simulink model "a3"  (R2021b)
settings: Solver=VariableStepAuto  StartTime=0.0  StopTime=500  RelTol=1e-3
libraries: simulink_extras x3
settings Model: Creator=郭义月  LastModifiedBy=郭义月

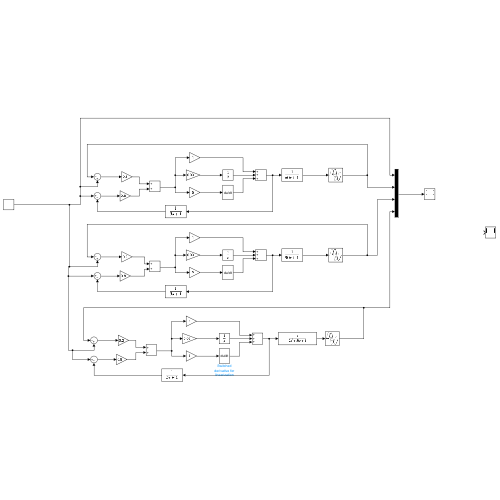
[thumbnail: Simulink's stored preview of the top-level diagram]
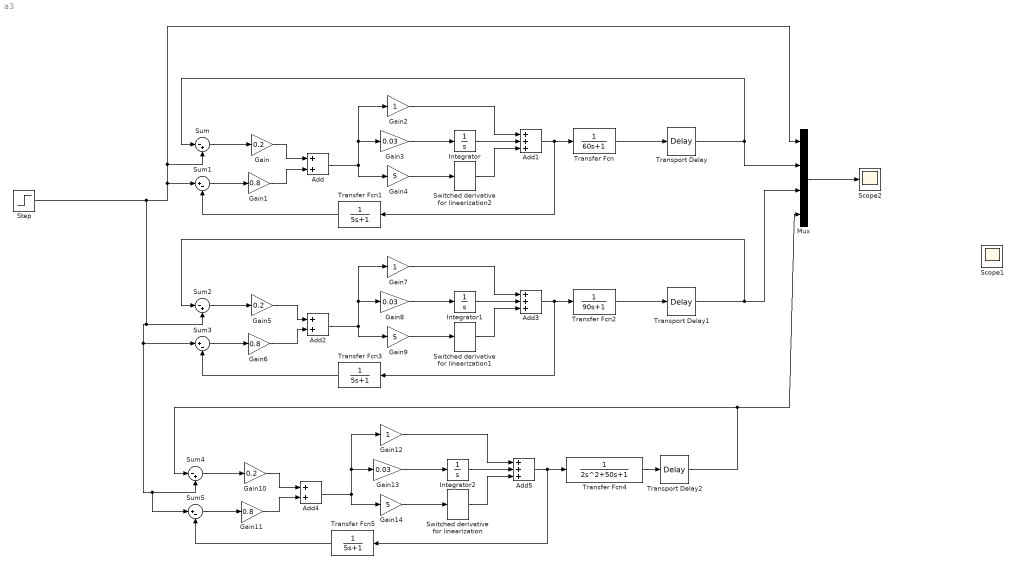
== system a3 ==
  Add : Sum
  Add1 : Sum  Inputs=+++
  Add2 : Sum
  Add3 : Sum  Inputs=+++
  Add4 : Sum
  Add5 : Sum  Inputs=+++
  Gain : Gain  Gain=0.2
  Gain1 : Gain  Gain=0.8
  Gain10 : Gain  Gain=0.2
  Gain11 : Gain  Gain=0.8
  Gain12 : Gain
  Gain13 : Gain  Gain=0.03
  Gain14 : Gain  Gain=5
  Gain2 : Gain
  Gain3 : Gain  Gain=0.03
  Gain4 : Gain  Gain=5
  Gain5 : Gain  Gain=0.2
  Gain6 : Gain  Gain=0.8
  Gain7 : Gain
  Gain8 : Gain  Gain=0.03
  Gain9 : Gain  Gain=5
  Integrator : Integrator
  Integrator1 : Integrator
  Integrator2 : Integrator
  Mux : Mux
  Scope1 : Scope
  Scope2 : Scope
  Step : Step  SampleTime=0
  Sum : Sum  Inputs=|-+
  Sum1 : Sum  Inputs=|+-
  Sum2 : Sum  Inputs=|-+
  Sum3 : Sum  Inputs=|+-
  Sum4 : Sum  Inputs=|-+
  Sum5 : Sum  Inputs=|+-
  Switched derivative for linearization : simulink_extras/Linearization/Switched derivative for linearization  switchVal=0  derivConst=100
      settings: SourceProductBaseCode=SL
  Switched derivative for linearization1 : simulink_extras/Linearization/Switched derivative for linearization  switchVal=0  derivConst=100
      settings: SourceProductBaseCode=SL
  Switched derivative for linearization2 : simulink_extras/Linearization/Switched derivative for linearization  switchVal=0  derivConst=100
      settings: SourceProductBaseCode=SL
  Transfer Fcn : TransferFcn  Denominator=[60 1]
  Transfer Fcn1 : TransferFcn  Denominator=[5 1]
  Transfer Fcn2 : TransferFcn  Denominator=[90 1]
  Transfer Fcn3 : TransferFcn  Denominator=[5 1]
  Transfer Fcn4 : TransferFcn  Denominator=[2 50 1]
  Transfer Fcn5 : TransferFcn  Denominator=[5 1]
  Transport Delay : TransportDelay  DelayTime=30
  Transport Delay1 : TransportDelay  DelayTime=30
  Transport Delay2 : TransportDelay  DelayTime=30
  wires:
  Sum/1 -> Gain/1
  Sum1/1 -> Gain1/1
  Gain/1 -> Add/1
  Gain1/1 -> Add/2
  Add/1 -> Gain4/1, Gain3/1, Gain2/1
  Gain3/1 -> Integrator/1
  Gain4/1 -> Switched derivative for linearization2/1
  Integrator/1 -> Add1/2
  Switched derivative for linearization2/1 -> Add1/3
  Add1/1 -> Transfer Fcn/1, Transfer Fcn1/1
  Transfer Fcn/1 -> Transport Delay/1
  Transfer Fcn1/1 -> Sum1/2
  Transport Delay/1 -> Sum/1, Mux/2
  Mux/1 -> Scope2/1
  Gain2/1 -> Add1/1
  Transfer Fcn3/1 -> Sum3/2
  Transport Delay1/1 -> Mux/3, Sum2/1
  Gain6/1 -> Add2/2
  Add3/1 -> Transfer Fcn2/1, Transfer Fcn3/1
  Gain9/1 -> Switched derivative for linearization1/1
  Gain7/1 -> Add3/1
  Sum2/1 -> Gain5/1
  Gain8/1 -> Integrator1/1
  Sum3/1 -> Gain6/1
  Gain5/1 -> Add2/1
  Add2/1 -> Gain9/1, Gain8/1, Gain7/1
  Switched derivative for linearization1/1 -> Add3/3
  Integrator1/1 -> Add3/2
  Transfer Fcn2/1 -> Transport Delay1/1
  Transfer Fcn5/1 -> Sum5/2
  Transport Delay2/1 -> Mux/4, Sum4/1
  Gain11/1 -> Add4/2
  Add5/1 -> Transfer Fcn4/1, Transfer Fcn5/1
  Step/1 -> Mux/1, Sum/2, Sum1/1, Sum2/2, Sum3/1, Sum5/1, Sum4/2
  Gain14/1 -> Switched derivative for linearization/1
  Gain12/1 -> Add5/1
  Sum4/1 -> Gain10/1
  Gain13/1 -> Integrator2/1
  Sum5/1 -> Gain11/1
  Gain10/1 -> Add4/1
  Add4/1 -> Gain14/1, Gain13/1, Gain12/1
  Switched derivative for linearization/1 -> Add5/3
  Integrator2/1 -> Add5/2
  Transfer Fcn4/1 -> Transport Delay2/1
